simulink model "k1vissrmt"  (Simulink 8.8)
settings: Solver=VariableStepAuto  StartTime=0.0  StopTime=10.0  RelTol=1e-3  EnableMultiTasking=on
libraries: cdsIPCx x10, cdsFilt x4, cdsCDO64 x3, cdsCDI64 x2, dac x2, TYPEB_MASTER x2, cdsAdcx0 x1, TOWER_MASTER x1, cdsParameters x1
settings Model: SuppressorTable=22 serialization::archive 11 0 3 0 0 0 11 0  Creator=controls  LastModifiedBy=controls
settings DataIOCC: SaveFormat=Dataset  SignalLoggingSaveFormat=Dataset
settings DebuggingCC: UnderspecifiedInitializationDetection=Simplified  MergeDetectMultiDrivingBlocksExec=error  FcnCallInpInsideContextMsg=error  AllowSymbolicDim=off  StateNameClashWarn=none
settings HardwareCC: ProdBitPerPointer=64  ProdBitPerSizeT=64  ProdBitPerPtrDiffT=64  ProdLargestAtomicFloat=Float  ProdIntDivRoundTo=Zero  ProdEndianess=LittleEndian  ProdWordSize=64  ProdHWDeviceType=Intel->x86-64 (Windows64)
settings GRTTargetCC: GeneratePreprocessorConditionals=Use local settings  CombineOutputUpdateFcns=on  GRTInterface=off

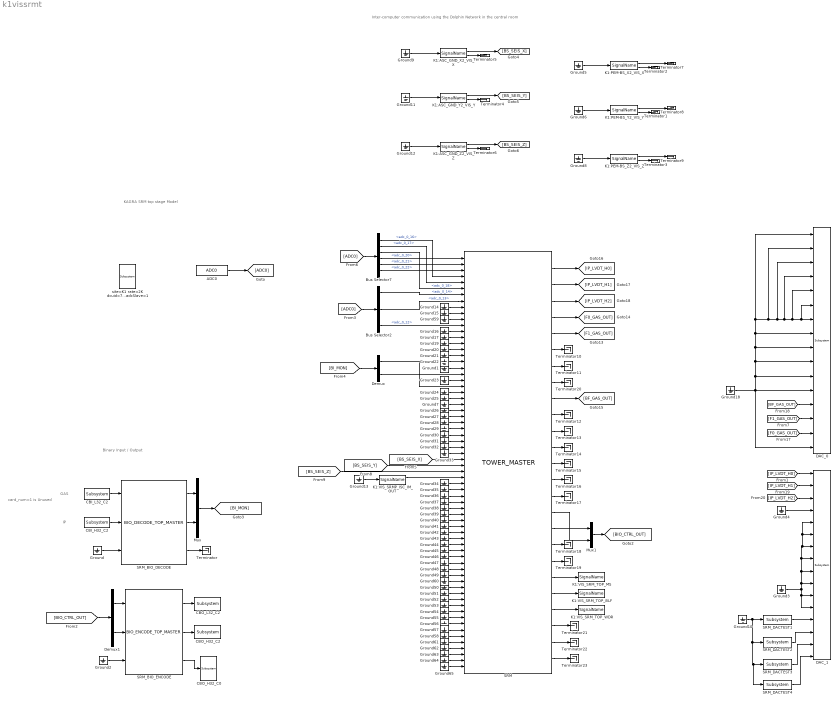
== system k1vissrmt ==
  note: KAGRA SRM top stage Model
  note: Binary Input / Output
  note: card_num=1 is Unused
  note: GAS
  note: IP
  note: Inter-computer communication using
      | the Dolphin Network in the central room
  ADC0 : cdsAdcx0/ADC0  Tag=cdsAdc  Description=|
      | type-GSC_16AI64SSA
      | card_num=0
      settings: AttributesFormatString=%<Description>\n%<Tag>
  Bus Selector2 : BusSelector  Description=ADC Selector  OutputSignals=adc_0_14,adc_0_13,adc_0_12
      settings: AttributesFormatString=%<Description>
  Bus Selector7 : BusSelector  Description=ADC Selector  OutputSignals=adc_0_16,adc_0_17,adc_0_18,adc_0_20,adc_0_21,adc_0_22
      settings: AttributesFormatString=%<Description>
  CBI_H32_C2 : cdsCDI64/Subsystem  Tag=cdsCDI64  Description=card_num=5
      settings: AttributesFormatString=%<Tag>\n%<Description>
  CBI_L32_C2 : cdsCDI64/Subsystem  Tag=cdsCDI64  Description=card_num=4
      settings: AttributesFormatString=%<Tag>\n%<Description>
  CBO_H32_C0 : cdsCDO64/Subsystem  Tag=cdsCDO64  Description=card_num=1
      settings: AttributesFormatString=%<Tag>\n%<Description>
  CBO_H32_C2 : cdsCDO64/Subsystem  Tag=cdsCDO64  Description=card_num=5
      settings: AttributesFormatString=%<Tag>\n%<Description>
  CBO_L32_C2 : cdsCDO64/Subsystem  Tag=cdsCDO64  Description=card_num=4
      settings: AttributesFormatString=%<Tag>\n%<Description>
  DAC_0 : dac/Subsystem  Description=|
      | type=GSC_16AO16,
      | card_num=0
      settings: AttributesFormatString=%<Description>
  DAC_1 : dac/Subsystem  Description=|
      | type=GSC_16AO16,
      | card_num=1
      settings: AttributesFormatString=%<Description>
  Demux : Demux  Outputs=2
  Demux1 : Demux  Outputs=2
  Ground{,1..65} (66 alike) : Ground
  K1:ASC_GND_X2_VIS_X : cdsIPCx/SignalName  Tag=cdsIPCx_PCIE  Description=Inter-Process Communication via PCI Express network.
      settings: AttributesFormatString=%<Tag>
  K1:ASC_GND_Y2_VIS_Y : cdsIPCx/SignalName  Tag=cdsIPCx_PCIE  Description=Inter-Process Communication via PCI Express network.
      settings: AttributesFormatString=%<Tag>
  K1:ASC_GND_Z2_VIS_Z : cdsIPCx/SignalName  Tag=cdsIPCx_PCIE  Description=Inter-Process Communication via PCI Express network.
      settings: AttributesFormatString=%<Tag>
  K1:PEM-BS_X2_VIS_X : cdsIPCx/SignalName  Tag=cdsIPCx_PCIE  Description=Inter-Process Communication via PCI Express network.
      settings: AttributesFormatString=%<Tag>
  K1:PEM-BS_Y2_VIS_Y : cdsIPCx/SignalName  Tag=cdsIPCx_PCIE  Description=Inter-Process Communication via PCI Express network.
      settings: AttributesFormatString=%<Tag>
  K1:PEM-BS_Z2_VIS_Z : cdsIPCx/SignalName  Tag=cdsIPCx_PCIE  Description=Inter-Process Communication via PCI Express network.
      settings: AttributesFormatString=%<Tag>
  K1:VIS_SRMP_ISC_IM_OUT : cdsIPCx/SignalName  Tag=cdsIPCx_SHMEM  Description=Inter-Process Communication via Shared memory.
      settings: AttributesFormatString=%<Tag>
  K1:VIS_SRM_TOP_BLF : cdsIPCx/SignalName  Tag=cdsIPCx_SHMEM  Description=Inter-Process Communication via Shared memory.
      settings: AttributesFormatString=%<Tag>
  K1:VIS_SRM_TOP_MS : cdsIPCx/SignalName  Tag=cdsIPCx_SHMEM  Description=Inter-Process Communication via Shared memory.
      settings: AttributesFormatString=%<Tag>
  K1:VIS_SRM_TOP_WDR : cdsIPCx/SignalName  Tag=cdsIPCx_SHMEM  Description=Inter-Process Communication via Shared memory.
      settings: AttributesFormatString=%<Tag>
  Mux : Mux  Inputs=2
  Mux1 : Mux  Inputs=2
  SRM : TOWER_MASTER/TOWER_MASTER
  SRM_BIO_DECODE : TYPEB_MASTER/BIO_DECODE_TOP_MASTER
  SRM_BIO_ENCODE : TYPEB_MASTER/BIO_ENCODE_TOP_MASTER
  SRM_DACTEST1 : cdsFilt/Subsystem  Tag=cdsFilt  Description=|
      | Purpose:                                                                                                                                                                                                                                  
      | Standard CDS IIR filter module.                                                                                                                                                                                                           
      |                                                                                                                                                                                                                                           
      | Operation:                                                                                                                                                                                                                                
      | Consists of 10 second order section IIR filters, plus a ramped gain stage. In FE code, also provides pre-defined test points and excitation channel inputs. The filter coefficients are defined in the LIGO system using the 'foton' tool.
      |                                                                                                                                                                                                                                           
      | Usage:                                                                                                                                                                                                                                    
      | Name the part with the desired filter module name.
      settings: AttributesFormatString=%<Tag>
  SRM_DACTEST2 : cdsFilt/Subsystem  Tag=cdsFilt  Description=|
      | Purpose:                                                                                                                                                                                                                                  
      | Standard CDS IIR filter module.                                                                                                                                                                                                           
      |                                                                                                                                                                                                                                           
      | Operation:                                                                                                                                                                                                                                
      | Consists of 10 second order section IIR filters, plus a ramped gain stage. In FE code, also provides pre-defined test points and excitation channel inputs. The filter coefficients are defined in the LIGO system using the 'foton' tool.
      |                                                                                                                                                                                                                                           
      | Usage:                                                                                                                                                                                                                                    
      | Name the part with the desired filter module name.
      settings: AttributesFormatString=%<Tag>
  SRM_DACTEST3 : cdsFilt/Subsystem  Tag=cdsFilt  Description=|
      | Purpose:                                                                                                                                                                                                                                  
      | Standard CDS IIR filter module.                                                                                                                                                                                                           
      |                                                                                                                                                                                                                                           
      | Operation:                                                                                                                                                                                                                                
      | Consists of 10 second order section IIR filters, plus a ramped gain stage. In FE code, also provides pre-defined test points and excitation channel inputs. The filter coefficients are defined in the LIGO system using the 'foton' tool.
      |                                                                                                                                                                                                                                           
      | Usage:                                                                                                                                                                                                                                    
      | Name the part with the desired filter module name.
      settings: AttributesFormatString=%<Tag>
  SRM_DACTEST4 : cdsFilt/Subsystem  Tag=cdsFilt  Description=|
      | Purpose:                                                                                                                                                                                                                                  
      | Standard CDS IIR filter module.                                                                                                                                                                                                           
      |                                                                                                                                                                                                                                           
      | Operation:                                                                                                                                                                                                                                
      | Consists of 10 second order section IIR filters, plus a ramped gain stage. In FE code, also provides pre-defined test points and excitation channel inputs. The filter coefficients are defined in the LIGO system using the 'foton' tool.
      |                                                                                                                                                                                                                                           
      | Usage:                                                                                                                                                                                                                                    
      | Name the part with the desired filter module name.
      settings: AttributesFormatString=%<Tag>
  Terminator{,1..23} (24 alike) : Terminator
  site=K1 rate=2K dcuid=75 host=k1srm specific_cpu=2 adcSlave=1 : cdsParameters/Subsystem  Tag=cdsParameters  Description=|
      | Purpose:                                                                                                                                                                                                                                
      | Provide system parameters to the FE code generator to properly configure the generated EPICS names, rep rate of the FE controller, and the Data Acquisition node ID for proper storage of data from this FE controller.                 
      |                                                                                                                                                                                                                                         
      | Useage:                                                                                                                                                                                                                                 
      | The part NAME field is used to identify the FE parameters. It must be of the form:                                                                                                                                                      
      | site=                                                                                                                                                                                                                                   
      | rate=                                                                                                                                                                                                                                   
      | dcuid=                                                                                                                                                                                                                                  
      |                                                                                                                                                                                                                                         
      | Where:                                                                                                                                                                                                                                  
      | site= argument may be H1, H2, L1, M1, G1, either as a single argument or multiple, for example site=H1,H2. These are the only names allowed. These will become the first two characters of all EPICS and signal names (for example G1:).
      |                                                                                                                                                                                                                                         
      | rate= may be 2K, 16K, 32K, or 64K                                                                                                                                                                                                       
      |                                                                                                                                                                                                                                         
      | dcuid= is site specific ie it must be unique at each site.
      settings: AttributesFormatString=%<Tag>
  wires:
  SRM/4 -> [F0_GAS_OUT]
  SRM/5 -> [F1_GAS_OUT]
  SRM/9 -> [BF_GAS_OUT]
  ADC0/1 -> [ADC0]
  [ADC0] -> Bus Selector7/1
  [ADC0] -> Bus Selector2/1
  Bus Selector2/2 -> SRM/8  "<adc_0_13>"
  Bus Selector2/3 -> SRM/12  "<adc_0_12>"
  Bus Selector7/1 -> SRM/4  "<adc_0_16>"
  Bus Selector7/2 -> SRM/5  "<adc_0_17>"
  Bus Selector7/3 -> SRM/6  "<adc_0_18>"
  Bus Selector7/4 -> SRM/1  "<adc_0_20>"
  Bus Selector7/5 -> SRM/2  "<adc_0_21>"
  Bus Selector7/6 -> SRM/3  "<adc_0_22>"
  Ground7/1 -> SRM/25
  [BI_MON] -> Demux/1
  Ground1/1 -> SRM/19
  Mux1/1 -> [BIO_CTRL_OUT]
  [F1_GAS_OUT] -> DAC_0/14
  [F0_GAS_OUT] -> DAC_0/15
  [BF_GAS_OUT] -> DAC_0/13
  SRM/2 -> [IP_LVDT_H1]
  SRM/1 -> [IP_LVDT_H0]
  SRM/3 -> [IP_LVDT_H2]
  [IP_LVDT_H0] -> DAC_1/1
  [IP_LVDT_H1] -> DAC_1/2
  [IP_LVDT_H2] -> DAC_1/3
  Bus Selector2/1 -> SRM/7  "<adc_0_14>"
  Ground18/1 -> DAC_0/11, DAC_0/10, DAC_0/9, DAC_0/1, DAC_0/2, DAC_0/3, DAC_0/4, DAC_0/5, DAC_0/6, DAC_0/7, DAC_0/8, DAC_0/16, DAC_0/12
  Ground3/1 -> DAC_1/12, DAC_1/11, DAC_1/5, DAC_1/6, DAC_1/7, DAC_1/8, DAC_1/9, DAC_1/10
  SRM_DACTEST3/1 -> DAC_1/15
  SRM_DACTEST4/1 -> DAC_1/16
  SRM_DACTEST2/1 -> DAC_1/14
  SRM_DACTEST1/1 -> DAC_1/13
  Ground10/1 -> SRM_DACTEST4/1, SRM_DACTEST3/1, SRM_DACTEST2/1, SRM_DACTEST1/1
  SRM/20 -> K1:VIS_SRM_TOP_MS/1
  SRM/22 -> K1:VIS_SRM_TOP_WDR/1
  SRM_BIO_ENCODE/1 -> CBO_L32_C2/1
  CBI_L32_C2/1 -> SRM_BIO_DECODE/1
  SRM_BIO_DECODE/1 -> Mux/1
  SRM_BIO_DECODE/2 -> Mux/2
  Mux/1 -> [BI_MON]
  [BIO_CTRL_OUT] -> Demux1/1
  CBI_H32_C2/1 -> SRM_BIO_DECODE/2
  SRM_BIO_ENCODE/2 -> CBO_H32_C2/1
  Demux1/2 -> SRM_BIO_ENCODE/2
  Ground/1 -> SRM_BIO_DECODE/3
  SRM_BIO_DECODE/3 -> Terminator/1
  Demux1/1 -> SRM_BIO_ENCODE/1
  SRM_BIO_ENCODE/3 -> CBO_H32_C0/1
  Ground2/1 -> SRM_BIO_ENCODE/3
  SRM/21 -> K1:VIS_SRM_TOP_BLF/1
  Ground4/1 -> DAC_1/4
  Ground5/1 -> K1:PEM-BS_X2_VIS_X/1
  Ground6/1 -> K1:PEM-BS_Y2_VIS_Y/1
  Ground8/1 -> K1:PEM-BS_Z2_VIS_Z/1
  K1:PEM-BS_X2_VIS_X/1 -> Terminator7/1
  K1:PEM-BS_Y2_VIS_Y/1 -> Terminator8/1
  K1:PEM-BS_Z2_VIS_Z/1 -> Terminator9/1
  K1:PEM-BS_X2_VIS_X/2 -> Terminator2/1
  K1:PEM-BS_Y2_VIS_Y/2 -> Terminator1/1
  K1:PEM-BS_Z2_VIS_Z/2 -> Terminator3/1
  [BS_SEIS_X] -> SRM/34
  [BS_SEIS_Z] -> SRM/36
  [BS_SEIS_Y] -> SRM/35
  Ground9/1 -> K1:ASC_GND_X2_VIS_X/1
  Ground11/1 -> K1:ASC_GND_Y2_VIS_Y/1
  Ground12/1 -> K1:ASC_GND_Z2_VIS_Z/1
  K1:ASC_GND_X2_VIS_X/1 -> [BS_SEIS_X]
  K1:ASC_GND_Y2_VIS_Y/1 -> [BS_SEIS_Y]
  K1:ASC_GND_Z2_VIS_Z/1 -> [BS_SEIS_Z]
  K1:ASC_GND_X2_VIS_X/2 -> Terminator5/1
  K1:ASC_GND_Y2_VIS_Y/2 -> Terminator4/1
  K1:ASC_GND_Z2_VIS_Z/2 -> Terminator6/1
  Ground13/1 -> K1:VIS_SRMP_ISC_IM_OUT/1
  K1:VIS_SRMP_ISC_IM_OUT/1 -> SRM/37
  SRM/16 -> Mux1/2
  SRM/17 -> Mux1/1
  Ground14/1 -> SRM/9
  Ground15/1 -> SRM/10
  Ground16/1 -> SRM/13
  Ground17/1 -> SRM/14
  Ground19/1 -> SRM/15
  Ground20/1 -> SRM/16
  Ground21/1 -> SRM/17
  Ground22/1 -> SRM/18
  Ground23/1 -> SRM/21
  Ground24/1 -> SRM/23
  Ground25/1 -> SRM/24
  Ground26/1 -> SRM/26
  Ground27/1 -> SRM/27
  Ground28/1 -> SRM/28
  Ground29/1 -> SRM/29
  Ground30/1 -> SRM/30
  Ground31/1 -> SRM/31
  Ground32/1 -> SRM/32
  Ground33/1 -> SRM/33
  Ground34/1 -> SRM/38
  Ground35/1 -> SRM/39
  Ground36/1 -> SRM/40
  Ground37/1 -> SRM/41
  Ground38/1 -> SRM/42
  Ground39/1 -> SRM/43
  Ground40/1 -> SRM/44
  Ground41/1 -> SRM/45
  Ground42/1 -> SRM/46
  Ground43/1 -> SRM/47
  Ground44/1 -> SRM/48
  Ground45/1 -> SRM/49
  Ground46/1 -> SRM/50
  Ground47/1 -> SRM/51
  Ground48/1 -> SRM/52
  Ground49/1 -> SRM/53
  Ground50/1 -> SRM/55
  Ground51/1 -> SRM/56
  Ground52/1 -> SRM/57
  Ground53/1 -> SRM/58
  Ground54/1 -> SRM/59
  Ground55/1 -> SRM/60
  Ground56/1 -> SRM/61
  Ground57/1 -> SRM/62
  Ground58/1 -> SRM/63
  SRM/6 -> Terminator10/1
  SRM/7 -> Terminator11/1
  SRM/10 -> Terminator12/1
  SRM/11 -> Terminator13/1
  SRM/13 -> Terminator15/1
  SRM/14 -> Terminator16/1
  SRM/15 -> Terminator17/1
  SRM/18 -> Terminator18/1
  SRM/19 -> Terminator19/1
  Demux/1 -> SRM/22
  Demux/2 -> SRM/20
  Ground59/1 -> SRM/11
  Ground60/1 -> SRM/54
  SRM/12 -> Terminator14/1
  SRM/8 -> Terminator20/1
  Ground63/1 -> SRM/66
  Ground62/1 -> SRM/65
  Ground61/1 -> SRM/64
  SRM/24 -> Terminator22/1
  SRM/23 -> Terminator21/1
  SRM/25 -> Terminator23/1
  Ground64/1 -> SRM/67
  Ground65/1 -> SRM/68
